simulink model "MOVH_Test"  (R2016a)
settings: Solver=FixedStepDiscrete  StartTime=0.0  StopTime=10.0  FixedStep=0.005  RelTol=1e-3
undefined symbols (not defined in the file): sigbuilder_block
libraries: MOVH x1
settings Model: Creator=oelkawok  LastModifiedBy=oelkawok

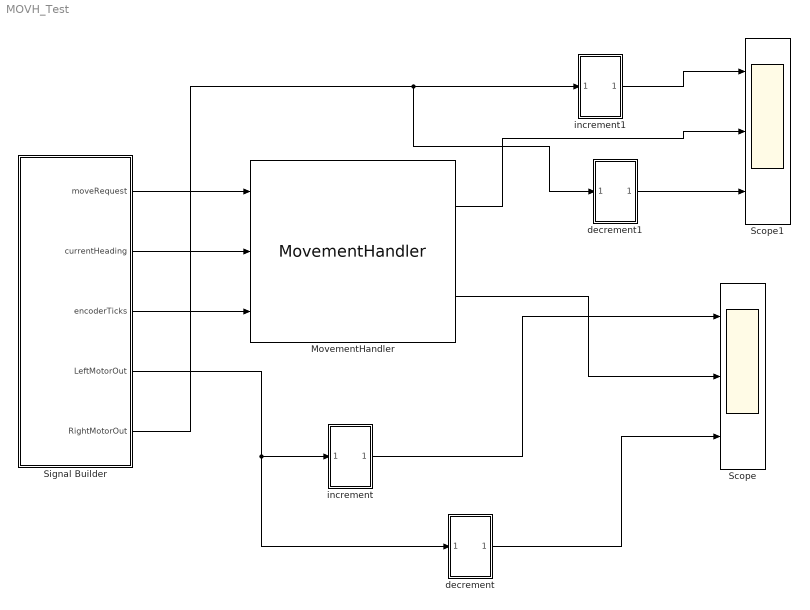
== system MOVH_Test ==
  MovementHandler : MOVH/MovementHandler
  Scope : Scope  NumInputPorts=3
  Scope1 : Scope  NumInputPorts=3
  Signal Builder : Subsystem  Tag=STV Subsys  LoadFcn=sigbuilder_block('load',[5.4 34.2 565.2 553.2 ]);  StartFcn=sigbuilder_block('start');  StopFcn=sigbuilder_block('stop');  ClipboardFcn=sigbuilder_block('clipboard');  mask(Sigbuilder block){}
      mask help: Simulink:masks:SigbuilderBlock_MD
      mask init:
      | if ~strcmp(get_param(bdroot(gcbh),'SimulationStatus'),'stopped') tuvar = sigbuilder_block('maskInit'); end
      settings: CopyFcn=sigbuilder_block('copy');  DeleteFcn=sigbuilder_block('delete');  ModelCloseFcn=sigbuilder_block('modelClose');  PreSaveFcn=sigbuilder_block('preSave');  PauseFcn=sigbuilder_block('pause');  ContinueFcn=sigbuilder_block('continue');  NameChangeFcn=sigbuilder_block('namechange');  OpenFcn=sigbuilder_block('open',[5.4 34.2 565.2 553.2 ]);  CloseFcn=sigbuilder_block('close');
      mask Display: plot(0, 0, 100, 100,[2, 2, 32, 32, 2], [68, 8, 8, 68, 68],[32, 2], [38, 38], [32, 19, 2],[53, 60, 44], [32, 17, 17, 2],[16, 16, 31, 31]);txt = getActiveGroup(gcbh);text(2, 100, txt,'verticalAlignment', 'top');
  decrement : Subsystem
  decrement1 : Subsystem
  increment : Subsystem
  increment1 : Subsystem
  wires:
  Signal Builder/2(currentHeading) -> MovementHandler/2
  Signal Builder/1(moveRequest) -> MovementHandler/1
  Signal Builder/3(encoderTicks) -> MovementHandler/3
  Signal Builder/4(LeftMotorOut) -> decrement/1(In1), increment/1(In1)
  MovementHandler/2 -> Scope/2
  increment/1(Out1) -> Scope/1
  decrement/1(Out1) -> Scope/3
  Signal Builder/5(RightMotorOut) -> decrement1/1(In1), increment1/1(In1)
  increment1/1(Out1) -> Scope1/1
  decrement1/1(Out1) -> Scope1/3
  MovementHandler/1 -> Scope1/2

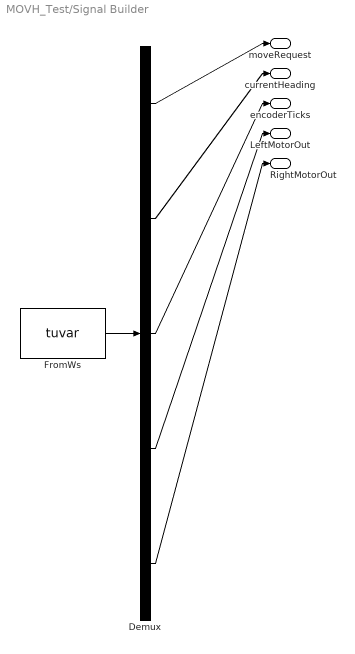
== system MOVH_Test/Signal Builder ==
  Demux : Demux  Tag=STV Demux  Outputs=5
  FromWs : FromWorkspace  Tag=STV FromWs  VariableName=tuvar  SampleTime=0
      SigBuilderData=|
      | common.afterFinalStr = 'Extrapolate'
      | common.sampleTime = 0
      | dataSet(1).timeRange = [0 10]
      | dataSet(1).name = 'TurnLeft_TurnRight'
      | dataSet(2).timeRange = [0 10]
      | dataSet(2).name = 'UTurnRight'
      | dataSet(3).timeRange = [0 10]
      | dataSet(3).name = 'UTurnLeft'
      | dataSet(4).timeRange = [0 10]
      | dataSet(4).name = 'UTurn_Stop'
      | sbobj.Groups(1).Name = 'TurnLeft_TurnRight'
      | sbobj.Groups(1).Signals(1).Name = 'moveRequest'
      | sbobj.Groups(1).Signals(1).XData = [0 2 2 4 4 6 6 8 8 10]
      | sbobj.Groups(1).Signals(1).YData = [20 20 1 1 21 21 1 1 2 2]
      | sbobj.Groups(1).Signals(2).Name = 'currentHeading'
      | sbobj.Groups(1).Signals(2).XData = [0 2 2 4 6 6 10]
      | sbobj.Groups(1).Signals(2).YData = [270 270 180 180 180 270 270]
      | sbobj.Groups(1).Signals(3).Name = 'encoderTicks'
      | sbobj.Groups(1).Signals(3).XData = [0 0.1 0.1 0.2 0.2 0.3 0.3 0.4 0.4 0.5 0.5 0.6 0.6 0.7 0.7 0.8 0.8 0.9 0.9 1 1 1.1 1.1 1.2 1.2 1.3 1.3 1.4 1.4 1.5 1.5 1.6 1.6 1.7 1.7 1.8 1.8 1.9 1.9 2 2 2.1 2.1 2.2 2.2 2.3 2.3 2.4 2.4 2.5 2.5 2.6 2.6 2.7 2.7 2.8 2.8 2.9 2.9 3 3 3.1 3.1 3.2 3.2 3.3 3.3 3.4 3.4 3.5 3.5 3.6 3.6 3.7 3.7 3.8 3.8 3.9 3.9 4 4 4.1 4.1 4.2 4.2 4.3 4.3 4.4 4.4 4.5 4.5 4.6 4.6 4.7 4.7 4.8 4.8 4.9 4.9 5 5 5.1 5.1 5.2 5.2 5.3 5.3 5.4 5.4 5.5 5.5 5.6 5.6 5.7 5.7 5.8 5.8 5.9 5.9 6 6 6.1 6.1 6.2 6.2 6.3 6.3 6.4 6.4 6.5 6.5 6.6 6.6 6.7 6.7 6.8 6.8 6.9 6.9 7 7 7.1 7.1 7.2 7.2 7.3 7.3 7.4 7.4 7.5 7.5 7.6 7.6 7.7 7.7 7.8 7.8 7.9 7.9 8 8 8.1 8.1 8.2 8.2 8.3 8.3 8.4 8.4 8.5 8.5 8.6 8.6 8.7 8.7 8.8 8.8 8.9 8.9 9 9 9.1 9.1 9.2 9.2 9.3 9.3 9.4 9.4 9.5 9.5 9.6 9.6 9.7 9.7 9.8 9.8 9.9 9.9 10]
      | sbobj.Groups(1).Signals(3).YData = [1000 1000 0 0 1000 1000 0 0 1000 1000 0 0 1000 1000 0 0 1000 1000 0 0 1000 1000 0 0 1000 1000 0 0 1000 1000 0 0 1000 1000 0 0 1000 1000 0 0 1000 1000 0 0 1000 1000 0 0 1000 1000 0 0 1000 1000 0 0 1000 1000 0 0 1000 1000 0 0 1000 1000 0 0 1000 1000 0 0 1000 1000 0 0 1000 1000 0 0 1000 1000 0 0 1000 1000 0 0 1000 1000 0 0 1000 1000 0 0 1000 1000 0 0 1000 1000 0 0 1000 1000 0 0 1000 1000 0 0 1000 1000 0 0 1000 1000 0 0 1000 1000 0 0 1000 1000 0 0 1000 1000 0 0 1000 1000 0 0 1000 1000 0 0 1000 1000 0 0 1000 1000 0 0 1000 1000 0 0 1000 1000 0 0 1000 1000 0 0 1000 1000 0 0 1000 1000 0 0 1000 1000 0 0 1000 1000 0 0 1000 1000 0 0 1000 1000 0 0 1000 1000 0 0 1000 1000 0 0 1000 1000 0 0 1000 1000 0 0]
      | sbobj.Groups(1).Signals(4).Name = 'LeftMotorOut'
      | sbobj.Groups(1).Signals(4).XData = [0 2 2 8 8 10]
      | sbobj.Groups(1).Signals(4).YData = [2 2 1 1 2 2]
      | sbobj.Groups(1).Signals(5).Name = 'RightMotorOut'
      | sbobj.Groups(1).Signals(5).XData = [0 2 4 4 6 6 8 8 10]
      | sbobj.Groups(1).Signals(5).YData = [1 1 1 2 2 1 1 2 2]
      | sbobj.Groups(2).Name = 'UTurnRight'
      | sbobj.Groups(2).Signals(1).Name = 'moveRequest'
      | sbobj.Groups(2).Signals(1).XData = [0 6 6 10]
      | sbobj.Groups(2).Signals(1).YData = [22 22 1 1]
      | sbobj.Groups(2).Signals(2).Name = 'currentHeading'
      | sbobj.Groups(2).Signals(2).XData = [0 2 2 5 6 6 10]
      | sbobj.Groups(2).Signals(2).YData = [270 270 0 0 0 90 90]
      | sbobj.Groups(2).Signals(3).Name = 'encoderTicks'
      | sbobj.Groups(2).Signals(3).XData = [0 0.1 0.1 0.2 0.2 0.3 0.3 0.4 0.4 0.5 0.5 0.6 0.6 0.7 0.7 0.8 0.8 0.9 0.9 1 1 1.1 1.1 1.2 1.2 1.3 1.3 1.4 1.4 1.5 1.5 1.6 1.6 1.7 1.7 1.8 1.8 1.9 1.9 2 2 2.1 2.1 2.2 2.2 2.3 2.3 2.4 2.4 2.5 2.5 2.6 2.6 2.7 2.7 2.8 2.8 2.9 2.9 3 3 3.1 3.1 3.2 3.2 3.3 3.3 3.4 3.4 3.5 3.5 3.6 3.6 3.7 3.7 3.8 3.8 3.9 3.9 4 4 4.1 4.1 4.2 4.2 4.3 4.3 4.4 4.4 4.5 4.5 4.6 4.6 4.7 4.7 4.8 4.8 4.9 4.9 5 5 5.1 5.1 5.2 5.2 5.3 5.3 5.4 5.4 5.5 5.5 5.6 5.6 5.7 5.7 5.8 5.8 5.9 5.9 6 6 6.1 6.1 6.2 6.2 6.3 6.3 6.4 6.4 6.5 6.5 6.6 6.6 6.7 6.7 6.8 6.8 6.9 6.9 7 7 7.1 7.1 7.2 7.2 7.3 7.3 7.4 7.4 7.5 7.5 7.6 7.6 7.7 7.7 7.8 7.8 7.9 7.9 8 8 8.1 8.1 8.2 8.2 8.3 8.3 8.4 8.4 8.5 8.5 8.6 8.6 8.7 8.7 8.8 8.8 8.9 8.9 9 9 9.1 9.1 9.2 9.2 9.3 9.3 9.4 9.4 9.5 9.5 9.6 9.6 9.7 9.7 9.8 9.8 9.9 9.9 10]
      | sbobj.Groups(2).Signals(3).YData = [1020 1020 0 0 1020 1020 0 0 1020 1020 0 0 1020 1020 0 0 1020 1020 0 0 1020 1020 0 0 1020 1020 0 0 1020 1020 0 0 1020 1020 0 0 1020 1020 0 0 1020 1020 0 0 1020 1020 0 0 1020 1020 0 0 1020 1020 0 0 1020 1020 0 0 1020 1020 0 0 1020 1020 0 0 1020 1020 0 0 1020 1020 0 0 1020 1020 0 0 1020 1020 0 0 1020 1020 0 0 1020 1020 0 0 1020 1020 0 0 1020 1020 0 0 1020 1020 0 0 1020 1020 0 0 1020 1020 0 0 1020 1020 0 0 1020 1020 0 0 1020 1020 0 0 1020 1020 0 0 1020 1020 0 0 1020 1020 0 0 1020 1020 0 0 1020 1020 0 0 1020 1020 0 0 1020 1020 0 0 1020 1020 0 0 1020 1020 0 0 1020 1020 0 0 1020 1020 0 0 1020 1020 0 0 1020 1020 0 0 1020 1020 0 0 1020 1020 0 0 1020 1020 0 0 1020 1020 0 0 1020 1020 0 0 1020 1020 0 0]
      | sbobj.Groups(2).Signals(4).Name = 'LeftMotorOut'
      | sbobj.Groups(2).Signals(4).XData = [0 4 6 10]
      | sbobj.Groups(2).Signals(4).YData = [1 1 1 1]
      | sbobj.Groups(2).Signals(5).Name = 'RightMotorOut'
      | sbobj.Groups(2).Signals(5).XData = [0 2 2 4.9 4.9 6 6 10]
      | sbobj.Groups(2).Signals(5).YData = [2 2 1 1 2 2 1 1]
      | sbobj.Groups(3).Name = 'UTurnLeft'
      | sbobj.Groups(3).Signals(1).Name = 'moveRequest'
      | sbobj.Groups(3).Signals(1).XData = [0 6 6 10]
      | sbobj.Groups(3).Signals(1).YData = [23 23 1 1]
      | sbobj.Groups(3).Signals(2).Name = 'currentHeading'
      | sbobj.Groups(3).Signals(2).XData = [0 2 2 6 6 10]
      | sbobj.Groups(3).Signals(2).YData = [270 270 180 180 90 90]
      | sbobj.Groups(3).Signals(3).Name = 'encoderTicks'
      | sbobj.Groups(3).Signals(3).XData = [0 0.1 0.1 0.2 0.2 0.3 0.3 0.4 0.4 0.5 0.5 0.6 0.6 0.7 0.7 0.8 0.8 0.9 0.9 1 1 1.1 1.1 1.2 1.2 1.3 1.3 1.4 1.4 1.5 1.5 1.6 1.6 1.7 1.7 1.8 1.8 1.9 1.9 2 2 2.1 2.1 2.2 2.2 2.3 2.3 2.4 2.4 2.5 2.5 2.6 2.6 2.7 2.7 2.8 2.8 2.9 2.9 3 3 3.1 3.1 3.2 3.2 3.3 3.3 3.4 3.4 3.5 3.5 3.6 3.6 3.7 3.7 3.8 3.8 3.9 3.9 4 4 4.1 4.1 4.2 4.2 4.3 4.3 4.4 4.4 4.5 4.5 4.6 4.6 4.7 4.7 4.8 4.8 4.9 4.9 5 5 5.1 5.1 5.2 5.2 5.3 5.3 5.4 5.4 5.5 5.5 5.6 5.6 5.7 5.7 5.8 5.8 5.9 5.9 6 6 6.1 6.1 6.2 6.2 6.3 6.3 6.4 6.4 6.5 6.5 6.6 6.6 6.7 6.7 6.8 6.8 6.9 6.9 7 7 7.1 7.1 7.2 7.2 7.3 7.3 7.4 7.4 7.5 7.5 7.6 7.6 7.7 7.7 7.8 7.8 7.9 7.9 8 8 8.1 8.1 8.2 8.2 8.3 8.3 8.4 8.4 8.5 8.5 8.6 8.6 8.7 8.7 8.8 8.8 8.9 8.9 9 9 9.1 9.1 9.2 9.2 9.3 9.3 9.4 9.4 9.5 9.5 9.6 9.6 9.7 9.7 9.8 9.8 9.9 9.9 10]
      | sbobj.Groups(3).Signals(3).YData = [1020 1020 0 0 1020 1020 0 0 1020 1020 0 0 1020 1020 0 0 1020 1020 0 0 1020 1020 0 0 1020 1020 0 0 1020 1020 0 0 1020 1020 0 0 1020 1020 0 0 1020 1020 0 0 1020 1020 0 0 1020 1020 0 0 1020 1020 0 0 1020 1020 0 0 1020 1020 0 0 1020 1020 0 0 1020 1020 0 0 1020 1020 0 0 1020 1020 0 0 1020 1020 0 0 1020 1020 0 0 1020 1020 0 0 1020 1020 0 0 1020 1020 0 0 1020 1020 0 0 1020 1020 0 0 1020 1020 0 0 1020 1020 0 0 1020 1020 0 0 1020 1020 0 0 1020 1020 0 0 1020 1020 0 0 1020 1020 0 0 1020 1020 0 0 1020 1020 0 0 1020 1020 0 0 1020 1020 0 0 1020 1020 0 0 1020 1020 0 0 1020 1020 0 0 1020 1020 0 0 1020 1020 0 0 1020 1020 0 0 1020 1020 0 0 1020 1020 0 0 1020 1020 0 0 1020 1020 0 0 1020 1020 0 0 1020 1020 0 0]
      | sbobj.Groups(3).Signals(4).Name = 'LeftMotorOut'
      | sbobj.Groups(3).Signals(4).XData = [0 2 2 5 5 6 6 10]
      | sbobj.Groups(3).Signals(4).YData = [2 2 1 1 2 2 1 1]
      | sbobj.Groups(3).Signals(5).Name = 'RightMotorOut'
      | sbobj.Groups(3).Signals(5).XData = [0 10]
      | sbobj.Groups(3).Signals(5).YData = [1 1]
      | sbobj.Groups(4).Name = 'UTurn_Stop'
      | sbobj.Groups(4).Signals(1).Name = 'moveRequest'
      | sbobj.Groups(4).Signals(1).XData = [0 3 3 6 6 8 8 10]
      | sbobj.Groups(4).Signals(1).YData = [24 24 1 1 5 5 1 1]
      | sbobj.Groups(4).Signals(2).Name = 'currentHeading'
      | sbobj.Groups(4).Signals(2).XData = [0 1.42 1.42 2.14 3 3 6 10]
      | sbobj.Groups(4).Signals(2).YData = [270 270 0 0 0 90 90 90]
      | sbobj.Groups(4).Signals(3).Name = 'encoderTicks'
      | sbobj.Groups(4).Signals(3).XData = [0 0.1 0.1 0.2 0.2 0.3 0.3 0.4 0.4 0.5 0.5 0.6 0.6 0.7 0.7 0.8 0.8 0.9 0.9 1 1 1.1 1.1 1.2 1.2 1.3 1.3 1.4 1.4 1.5 1.5 1.6 1.6 1.7 1.7 1.8 1.8 1.9 1.9 2 2 2.1 2.1 2.2 2.2 2.3 2.3 2.4 2.4 2.5 2.5 2.6 2.6 2.7 2.7 2.8 2.8 2.9 2.9 3 3 3.1 3.1 3.2 3.2 3.3 3.3 3.4 3.4 3.5 3.5 3.6 3.6 3.7 3.7 3.8 3.8 3.9 3.9 4 4 4.1 4.1 4.2 4.2 4.3 4.3 4.4 4.4 4.5 4.5 4.6 4.6 4.7 4.7 4.8 4.8 4.9 4.9 5 5 5.1 5.1 5.2 5.2 5.3 5.3 5.4 5.4 5.5 5.5 5.6 5.6 5.7 5.7 5.8 5.8 5.9 5.9 6 8 8 8.1 8.1 8.2 8.2 8.3 8.3 8.4 8.4 8.5 8.5 8.6 8.6 8.7 8.7 8.8 8.8 8.9 8.9 9 9 9.1 9.1 9.2 9.2 9.3 9.3 9.4 9.4 9.5 9.5 9.6 9.6 9.7 9.7 9.8 9.8 9.9 9.9 10]
      | sbobj.Groups(4).Signals(3).YData = [1020 1020 0 0 1020 1020 0 0 1020 1020 0 0 1020 1020 0 0 1020 1020 0 0 1020 1020 0 0 1020 1020 0 0 1020 1020 0 0 1020 1020 0 0 1020 1020 0 0 1020 1020 0 0 1020 1020 0 0 1020 1020 0 0 1020 1020 0 0 1020 1020 0 0 1020 1020 0 0 1020 1020 0 0 1020 1020 0 0 1020 1020 0 0 1020 1020 0 0 1020 1020 0 0 1020 1020 0 0 1020 1020 0 0 1020 1020 0 0 1020 1020 0 0 1020 1020 0 0 1020 1020 0 0 1020 1020 0 0 1020 1020 0 0 1020 1020 0 0 0 1020 1020 0 0 1020 1020 0 0 1020 1020 0 0 1020 1020 0 0 1020 1020 0 0 1020 1020 0 0 1020 1020 0 0 1020 1020 0 0 1020 1020 0 0 1020 1020 0 0]
      | sbobj.Groups(4).Signals(4).Name = 'LeftMotorOut'
      | sbobj.Groups(4).Signals(4).XData = [0 2 5 6 6 8 8 10]
      | sbobj.Groups(4).Signals(4).YData = [1 1 1 1 5 5 1 1]
      | sbobj.Groups(4).Signals(5).Name = 'RightMotorOut'
      | sbobj.Groups(4).Signals(5).XData = [0 3 3 5 6 6 8 8 10]
      | sbobj.Groups(4).Signals(5).YData = [2 2 1 1 1 5 5 1 1]
  moveRequest : Outport  Tag=STV Outport
  currentHeading : Outport  Tag=STV Outport  Port=2
  encoderTicks : Outport  Tag=STV Outport  Port=3
  LeftMotorOut : Outport  Tag=STV Outport  Port=4
  RightMotorOut : Outport  Tag=STV Outport  Port=5
  wires:
  FromWs/1 -> Demux/1
  Demux/1 -> moveRequest/1
  Demux/2 -> currentHeading/1
  Demux/3 -> encoderTicks/1
  Demux/4 -> LeftMotorOut/1
  Demux/5 -> RightMotorOut/1

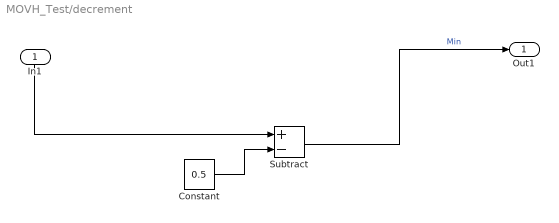
== system MOVH_Test/decrement ==
  In1 : Inport
  Constant : Constant  Value=0.5
  Subtract : Sum  Inputs=+-
  Out1 : Outport
  wires:
  Subtract/1 -> Out1/1  "Min"
  In1/1 -> Subtract/1
  Constant/1 -> Subtract/2

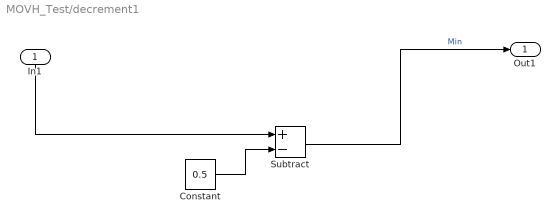
== system MOVH_Test/decrement1 ==
  In1 : Inport
  Constant : Constant  Value=0.5
  Subtract : Sum  Inputs=+-
  Out1 : Outport
  wires:
  Constant/1 -> Subtract/2
  In1/1 -> Subtract/1
  Subtract/1 -> Out1/1  "Min"

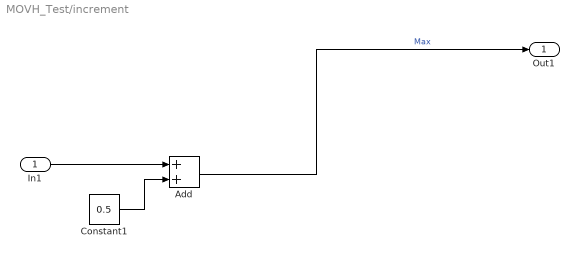
== system MOVH_Test/increment ==
  In1 : Inport
  Add : Sum
  Constant1 : Constant  Value=0.5
  Out1 : Outport
  wires:
  Constant1/1 -> Add/2
  Add/1 -> Out1/1  "Max"
  In1/1 -> Add/1

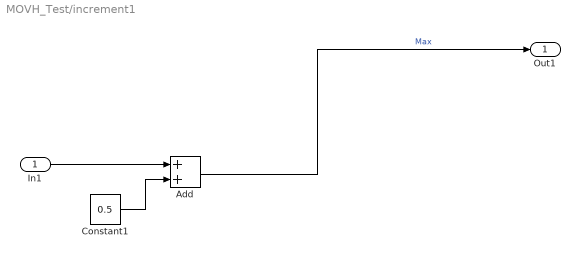
== system MOVH_Test/increment1 ==
  In1 : Inport
  Add : Sum
  Constant1 : Constant  Value=0.5
  Out1 : Outport
  wires:
  In1/1 -> Add/1
  Add/1 -> Out1/1  "Max"
  Constant1/1 -> Add/2
